simulink model "ALL_JP360_DBW_V6_5_1103"  (R2022a)
settings: Solver=FixedStepAuto  StartTime=0.0  StopTime=inf  FixedStep=0.01  RelTol=1e-3  EnableMultiTasking=on
model workspace (MAT data in the model file):
  g = 9.8
undefined symbols (not defined in the file or in its folder): canChannel, delta_v_p, IPM_Line_C0, IPM_Line_C1, IPM_Line_C2, IPM_Line_C3, M, M_p, MRR_ObjDistX, MRR_ObjDistY, MRR_ObjFusionCamID, MRR_ObjFusionSig, MRR_ObjID, MRR_ObjRelVelX, MRR_ObjRelVelY, MRR_ObjType, MRR_ObjUpdFlg, none, obj_vaild, untracktime, V, videoinput
libraries: canfdmsglib x230, canfdlib x76, slpidlib x24, simulink x18, dspstat3 x14, ctrlSharedLib x1, simulink_extras x1, imaqlib x1, realtime_pacer_lib x1, dspvision x1, visionsinks x1
(part 18 of 55)

== system ALL_JP360_DBW_V6_5_1103/MsgFromCAN/SRR_ADCU_MsgFromCAN/SRR_ADCU_FLR_OBJPos13_0x19D ==
  SRR_ADCU_FLR_OBJPos13_0x19DFromInData : Inport  OutDataTypeStr=Bus:CAN_FD_MESSAGE_BUS
  Bus Creator : BusCreator  Inputs=42  OutDataTypeStr=Bus:SRR_ADCU_FLR_OBJPos13_0x19D  NonVirtualBus=on
  CAN FD Unpack : canfdmsglib/CAN FD Unpack  CANdbFile=V363 SRR Private CAN-V1.3.dbc  MsgList=(none)  MsgName=FLR_OBJPos13_0x19D  ProtocolMode=CAN FD  MsgIDType=Standard (11-bit identifier)  MsgIdentifier=413  MsgLength=48  SignalInfo={'FLR_CRCCheck_0x19D','376','16','BE','unsigned','Standard','0','1','0','0','65535';'FLR_OBJ25_Dx','79','13','BE','unsigned','Standard','0','0.0625','-256','-256','255.938';'FLR_OBJ25_Dy','60','11','BE','unsigned','Standard','0','0.125','-128','-128','127.875';'FLR_OBJ25_ExistProb','112','6','BE','unsigned','Standard','0','2','0','0','100';'FLR_OBJ25_HeadingAngle','55','10','BE','unsigned','Standard','0','0.01','-3.14','-3.14','3.14';'FLR_OBJ25_Height','26','9','BE','unsigned','Standard','0','0.01','0','0','5.11';'FLR_OBJ25_Length','33','9','BE','unsigned','Standard','0','0.05','0','0','25.5';'FLR_OBJ25_Measured','126','2','BE','unsigned','Standard','0','1','0','0','3';'FLR_OBJ25_Motion_Status','162','3','BE','unsigned','Standard','0','1','0','0','7';'FLR_OBJ25_ObstacleProb','120','6','BE','unsigned','Standard','0','2','0','0','100';'FLR_OBJ25_RefPointDx','144','13','BE','unsigned','Standard','0','0.0625','-256','-256','255.938';'FLR_OBJ25_RefPointDy','141','11','BE','unsigned','Standard','0','0.125','-128','-128','127.875';'FLR_OBJ25_RefPointLoc','157','3','BE','unsigned','Standard','0','1','0','0','7';'FLR_OBJ25_RelAx','118','9','BE','unsigned','Standard','0','0.0625','-16','-16','15.9375';'FLR_OBJ25_RelAy','111','10','BE','unsigned','Standard','0','0.03125','-16','-16','15.9688';'FLR_OBJ25_RelVx','89','12','BE','unsigned','Standard','0','0.0625','-128','-128','127.938';'FLR_OBJ25_RelVy','85','10','BE','unsigned','Standard','0','0.125','-64','-64','63.875';'FLR_OBJ25_Track_Age','165','8','BE','unsigned','Standard','0','1','0','0','255';'FLR_OBJ25_Track_ID','1','7','BE','unsigned','Standard','0','1','0','0','127';'FLR_OBJ25_Type','14','3','BE','unsigned','Standard','0','1','0','0','7';'FLR_OBJ25_Width','19','11','BE','unsigned','Standard','0','0.01','0','0','12';'FLR_OBJ26_Dx','247','13','BE','unsigned','Standard','0','0.0625','-256','-256','255.938';'FLR_OBJ26_Dy','228','11','BE','unsigned','Standard','0','0.125','-128','-128','127.875';'FLR_OBJ26_ExistProb','280','6','BE','unsigned','Standard','0','2','0','0','100';'FLR_OBJ26_HeadingAngle','223','10','BE','unsigned','Standard','0','0.01','-3.14','-3.14','3.14';'FLR_OBJ26_Height','194','9','BE','unsigned','Standard','0','0.01','0','0','5.11';'FLR_OBJ26_Length','201','9','BE','unsigned','Standard','0','0.05','0','0','25.5';'FLR_OBJ26_Measured','294','2','BE','unsigned','Standard','0','1','0','0','3';'FLR_OBJ26_Motion_Status','330','3','BE','unsigned','Standard','0','1','0','0','7';'FLR_OBJ26_ObstacleProb','288','6','BE','unsigned','Standard','0','2','0','0','100';'FLR_OBJ26_RefPointDx','312','13','BE','unsigned','Standard','0','0.0625','-256','-256','255.938';'FLR_OBJ26_RefPointDy','309','11','BE','unsigned','Standard','0','0.125','-128','-128','127.875';'FLR_OBJ26_RefPointLoc','325','3','BE','unsigned','Standard','0','1','0','0','7';'FLR_OBJ26_RelAx','286','9','BE','unsigned','Standard','0','0.0625','-16','-16','15.9375';'FLR_OBJ26_RelAy','279','10','BE','unsigned','Standard','0','0.03125','-16','-16','15.9688';'FLR_OBJ26_RelVx','257','12','BE','unsigned','Standard','0','0.0625','-128','-128','127.938';'FLR_OBJ26_RelVy','253','10','BE','unsigned','Standard','0','0.125','-64','-64','63.875';'FLR_OBJ26_Track_Age','333','8','BE','unsigned','Standard','0','1','0','0','255';'FLR_OBJ26_Track_ID','169','7','BE','unsigned','Standard','0','1','0','0','127';'FLR_OBJ26_Type','182','3','BE','unsigned','Standard','0','1','0','0','7';'FLR_OBJ26_Width','187','11','BE','unsigned','Standard','0','0.01','0','0','12';'FLR_RollingCounter_0x19D','360','4','BE','unsigned','Standard','0','1','0','0','15'}  IDPort=off  TimestampPort=off  ErrorPort=off  RemotePort=off  LengthPort=off  StatusPort=off  BRSPort=off  ESIPort=off  DLCPort=off  ApplyMinMax=off
      settings: SourceProductBaseCode=ME,XP,VN  DataFormat=CANdb specified signals
  Data Type Conversion1 : DataTypeConversion  OutDataTypeStr=uint16  SaturateOnIntegerOverflow=off  RndMeth=Floor
  Data Type Conversion{4,8..10,13,19..20,24,28..30,33,39..40,42} (15 alike) : DataTypeConversion  OutDataTypeStr=int8  SaturateOnIntegerOverflow=off  RndMeth=Floor
  Data Type Conversion{2..3,5..7,11..12,14..17,21..23,25..27,31..32,34..37,41} (24 alike) : DataTypeConversion  OutDataTypeStr=single  SaturateOnIntegerOverflow=off  RndMeth=Floor
  Data Type Conversion18 : DataTypeConversion  OutDataTypeStr=uint8  SaturateOnIntegerOverflow=off  RndMeth=Floor
  Data Type Conversion38 : DataTypeConversion  OutDataTypeStr=uint8  SaturateOnIntegerOverflow=off  RndMeth=Floor
  SRR_ADCU_FLR_OBJPos13_0x19DFromOutData : Outport  OutDataTypeStr=Bus:SRR_ADCU_FLR_OBJPos13_0x19D
  wires:
  CAN FD Unpack/1 -> Data Type Conversion1/1
  CAN FD Unpack/2 -> Data Type Conversion2/1
  CAN FD Unpack/3 -> Data Type Conversion3/1
  CAN FD Unpack/4 -> Data Type Conversion4/1
  CAN FD Unpack/5 -> Data Type Conversion5/1
  CAN FD Unpack/6 -> Data Type Conversion6/1
  CAN FD Unpack/7 -> Data Type Conversion7/1
  CAN FD Unpack/8 -> Data Type Conversion8/1
  CAN FD Unpack/9 -> Data Type Conversion9/1
  CAN FD Unpack/10 -> Data Type Conversion10/1
  CAN FD Unpack/11 -> Data Type Conversion11/1
  CAN FD Unpack/12 -> Data Type Conversion12/1
  CAN FD Unpack/13 -> Data Type Conversion13/1
  CAN FD Unpack/14 -> Data Type Conversion14/1
  CAN FD Unpack/15 -> Data Type Conversion15/1
  CAN FD Unpack/16 -> Data Type Conversion16/1
  CAN FD Unpack/17 -> Data Type Conversion17/1
  CAN FD Unpack/18 -> Data Type Conversion18/1
  CAN FD Unpack/19 -> Data Type Conversion19/1
  CAN FD Unpack/20 -> Data Type Conversion20/1
  CAN FD Unpack/21 -> Data Type Conversion21/1
  CAN FD Unpack/22 -> Data Type Conversion22/1
  CAN FD Unpack/23 -> Data Type Conversion23/1
  CAN FD Unpack/24 -> Data Type Conversion24/1
  CAN FD Unpack/25 -> Data Type Conversion25/1
  CAN FD Unpack/26 -> Data Type Conversion26/1
  CAN FD Unpack/27 -> Data Type Conversion27/1
  CAN FD Unpack/28 -> Data Type Conversion28/1
  CAN FD Unpack/29 -> Data Type Conversion29/1
  CAN FD Unpack/30 -> Data Type Conversion30/1
  CAN FD Unpack/31 -> Data Type Conversion31/1
  CAN FD Unpack/32 -> Data Type Conversion32/1
  CAN FD Unpack/33 -> Data Type Conversion33/1
  CAN FD Unpack/34 -> Data Type Conversion34/1
  CAN FD Unpack/35 -> Data Type Conversion35/1
  CAN FD Unpack/36 -> Data Type Conversion36/1
  CAN FD Unpack/37 -> Data Type Conversion37/1
  CAN FD Unpack/38 -> Data Type Conversion38/1
  CAN FD Unpack/39 -> Data Type Conversion39/1
  CAN FD Unpack/40 -> Data Type Conversion40/1
  CAN FD Unpack/41 -> Data Type Conversion41/1
  CAN FD Unpack/42 -> Data Type Conversion42/1
  Data Type Conversion1/1 -> Bus Creator/1  "FLR_CRCCheck_0x19D"
  Data Type Conversion2/1 -> Bus Creator/2  "FLR_OBJ25_Dx"
  Data Type Conversion3/1 -> Bus Creator/3  "FLR_OBJ25_Dy"
  Data Type Conversion4/1 -> Bus Creator/4  "FLR_OBJ25_ExistProb"
  Data Type Conversion5/1 -> Bus Creator/5  "FLR_OBJ25_HeadingAngle"
  Data Type Conversion6/1 -> Bus Creator/6  "FLR_OBJ25_Height"
  Data Type Conversion7/1 -> Bus Creator/7  "FLR_OBJ25_Length"
  Data Type Conversion8/1 -> Bus Creator/8  "FLR_OBJ25_Measured"
  Data Type Conversion9/1 -> Bus Creator/9  "FLR_OBJ25_Motion_Status"
  Data Type Conversion10/1 -> Bus Creator/10  "FLR_OBJ25_ObstacleProb"
  Data Type Conversion11/1 -> Bus Creator/11  "FLR_OBJ25_RefPointDx"
  Data Type Conversion12/1 -> Bus Creator/12  "FLR_OBJ25_RefPointDy"
  Data Type Conversion13/1 -> Bus Creator/13  "FLR_OBJ25_RefPointLoc"
  Data Type Conversion14/1 -> Bus Creator/14  "FLR_OBJ25_RelAx"
  Data Type Conversion15/1 -> Bus Creator/15  "FLR_OBJ25_RelAy"
  Data Type Conversion16/1 -> Bus Creator/16  "FLR_OBJ25_RelVx"
  Data Type Conversion17/1 -> Bus Creator/17  "FLR_OBJ25_RelVy"
  Data Type Conversion18/1 -> Bus Creator/18  "FLR_OBJ25_Track_Age"
  Data Type Conversion19/1 -> Bus Creator/19  "FLR_OBJ25_Track_ID"
  Data Type Conversion20/1 -> Bus Creator/20  "FLR_OBJ25_Type"
  Data Type Conversion21/1 -> Bus Creator/21  "FLR_OBJ25_Width"
  Data Type Conversion22/1 -> Bus Creator/22  "FLR_OBJ26_Dx"
  Data Type Conversion23/1 -> Bus Creator/23  "FLR_OBJ26_Dy"
  Data Type Conversion24/1 -> Bus Creator/24  "FLR_OBJ26_ExistProb"
  Data Type Conversion25/1 -> Bus Creator/25  "FLR_OBJ26_HeadingAngle"
  Data Type Conversion26/1 -> Bus Creator/26  "FLR_OBJ26_Height"
  Data Type Conversion27/1 -> Bus Creator/27  "FLR_OBJ26_Length"
  Data Type Conversion28/1 -> Bus Creator/28  "FLR_OBJ26_Measured"
  Data Type Conversion29/1 -> Bus Creator/29  "FLR_OBJ26_Motion_Status"
  Data Type Conversion30/1 -> Bus Creator/30  "FLR_OBJ26_ObstacleProb"
  Data Type Conversion31/1 -> Bus Creator/31  "FLR_OBJ26_RefPointDx"
  Data Type Conversion32/1 -> Bus Creator/32  "FLR_OBJ26_RefPointDy"
  Data Type Conversion33/1 -> Bus Creator/33  "FLR_OBJ26_RefPointLoc"
  Data Type Conversion34/1 -> Bus Creator/34  "FLR_OBJ26_RelAx"
  Data Type Conversion35/1 -> Bus Creator/35  "FLR_OBJ26_RelAy"
  Data Type Conversion36/1 -> Bus Creator/36  "FLR_OBJ26_RelVx"
  Data Type Conversion37/1 -> Bus Creator/37  "FLR_OBJ26_RelVy"
  Data Type Conversion38/1 -> Bus Creator/38  "FLR_OBJ26_Track_Age"
  Data Type Conversion39/1 -> Bus Creator/39  "FLR_OBJ26_Track_ID"
  Data Type Conversion40/1 -> Bus Creator/40  "FLR_OBJ26_Type"
  Data Type Conversion41/1 -> Bus Creator/41  "FLR_OBJ26_Width"
  Data Type Conversion42/1 -> Bus Creator/42  "FLR_RollingCounter_0x19D"
  Bus Creator/1 -> SRR_ADCU_FLR_OBJPos13_0x19DFromOutData/1  "SRR_ADCU_FLR_OBJPos13_0x19DFromOutData"
  SRR_ADCU_FLR_OBJPos13_0x19DFromInData/1 -> CAN FD Unpack/1  "SRR_ADCU_FLR_OBJPos13_0x19DFromInData"

== system ALL_JP360_DBW_V6_5_1103/MsgFromCAN/SRR_ADCU_MsgFromCAN/SRR_ADCU_FLR_OBJPos14_0x19E ==
  SRR_ADCU_FLR_OBJPos14_0x19EFromInData : Inport  OutDataTypeStr=Bus:CAN_FD_MESSAGE_BUS
  Bus Creator : BusCreator  Inputs=42  OutDataTypeStr=Bus:SRR_ADCU_FLR_OBJPos14_0x19E  NonVirtualBus=on
  CAN FD Unpack : canfdmsglib/CAN FD Unpack  CANdbFile=V363 SRR Private CAN-V1.3.dbc  MsgList=(none)  MsgName=FLR_OBJPos14_0x19E  ProtocolMode=CAN FD  MsgIDType=Standard (11-bit identifier)  MsgIdentifier=414  MsgLength=48  SignalInfo={'FLR_CRCCheck_0x19E','376','16','BE','unsigned','Standard','0','1','0','0','65535';'FLR_OBJ27_Dx','79','13','BE','unsigned','Standard','0','0.0625','-256','-256','255.938';'FLR_OBJ27_Dy','60','11','BE','unsigned','Standard','0','0.125','-128','-128','127.875';'FLR_OBJ27_ExistProb','112','6','BE','unsigned','Standard','0','2','0','0','100';'FLR_OBJ27_HeadingAngle','55','10','BE','unsigned','Standard','0','0.01','-3.14','-3.14','3.14';'FLR_OBJ27_Height','26','9','BE','unsigned','Standard','0','0.01','0','0','5.11';'FLR_OBJ27_Length','33','9','BE','unsigned','Standard','0','0.05','0','0','25.5';'FLR_OBJ27_Measured','126','2','BE','unsigned','Standard','0','1','0','0','3';'FLR_OBJ27_Motion_Status','162','3','BE','unsigned','Standard','0','1','0','0','7';'FLR_OBJ27_ObstacleProb','120','6','BE','unsigned','Standard','0','2','0','0','100';'FLR_OBJ27_RefPointDx','144','13','BE','unsigned','Standard','0','0.0625','-256','-256','255.938';'FLR_OBJ27_RefPointDy','141','11','BE','unsigned','Standard','0','0.125','-128','-128','127.875';'FLR_OBJ27_RefPointLoc','157','3','BE','unsigned','Standard','0','1','0','0','7';'FLR_OBJ27_RelAx','118','9','BE','unsigned','Standard','0','0.0625','-16','-16','15.9375';'FLR_OBJ27_RelAy','111','10','BE','unsigned','Standard','0','0.03125','-16','-16','15.9688';'FLR_OBJ27_RelVx','89','12','BE','unsigned','Standard','0','0.0625','-128','-128','127.938';'FLR_OBJ27_RelVy','85','10','BE','unsigned','Standard','0','0.125','-64','-64','63.875';'FLR_OBJ27_Track_Age','165','8','BE','unsigned','Standard','0','1','0','0','255';'FLR_OBJ27_Track_ID','1','7','BE','unsigned','Standard','0','1','0','0','127';'FLR_OBJ27_Type','14','3','BE','unsigned','Standard','0','1','0','0','7';'FLR_OBJ27_Width','19','11','BE','unsigned','Standard','0','0.01','0','0','12';'FLR_OBJ28_Dx','247','13','BE','unsigned','Standard','0','0.0625','-256','-256','255.938';'FLR_OBJ28_Dy','228','11','BE','unsigned','Standard','0','0.125','-128','-128','127.875';'FLR_OBJ28_ExistProb','280','6','BE','unsigned','Standard','0','2','0','0','100';'FLR_OBJ28_HeadingAngle','223','10','BE','unsigned','Standard','0','0.01','-3.14','-3.14','3.14';'FLR_OBJ28_Height','194','9','BE','unsigned','Standard','0','0.01','0','0','5.11';'FLR_OBJ28_Length','201','9','BE','unsigned','Standard','0','0.05','0','0','25.5';'FLR_OBJ28_Measured','294','2','BE','unsigned','Standard','0','1','0','0','3';'FLR_OBJ28_Motion_Status','330','3','BE','unsigned','Standard','0','1','0','0','7';'FLR_OBJ28_ObstacleProb','288','6','BE','unsigned','Standard','0','2','0','0','100';'FLR_OBJ28_RefPointDx','312','13','BE','unsigned','Standard','0','0.0625','-256','-256','255.938';'FLR_OBJ28_RefPointDy','309','11','BE','unsigned','Standard','0','0.125','-128','-128','127.875';'FLR_OBJ28_RefPointLoc','325','3','BE','unsigned','Standard','0','1','0','0','7';'FLR_OBJ28_RelAx','286','9','BE','unsigned','Standard','0','0.0625','-16','-16','15.9375';'FLR_OBJ28_RelAy','279','10','BE','unsigned','Standard','0','0.03125','-16','-16','15.9688';'FLR_OBJ28_RelVx','257','12','BE','unsigned','Standard','0','0.0625','-128','-128','127.938';'FLR_OBJ28_RelVy','253','10','BE','unsigned','Standard','0','0.125','-64','-64','63.875';'FLR_OBJ28_Track_Age','333','8','BE','unsigned','Standard','0','1','0','0','255';'FLR_OBJ28_Track_ID','169','7','BE','unsigned','Standard','0','1','0','0','127';'FLR_OBJ28_Type','182','3','BE','unsigned','Standard','0','1','0','0','7';'FLR_OBJ28_Width','187','11','BE','unsigned','Standard','0','0.01','0','0','12';'FLR_RollingCounter_0x19E','360','4','BE','unsigned','Standard','0','1','0','0','15'}  IDPort=off  TimestampPort=off  ErrorPort=off  RemotePort=off  LengthPort=off  StatusPort=off  BRSPort=off  ESIPort=off  DLCPort=off  ApplyMinMax=off
      settings: SourceProductBaseCode=ME,XP,VN  DataFormat=CANdb specified signals
  Data Type Conversion1 : DataTypeConversion  OutDataTypeStr=uint16  SaturateOnIntegerOverflow=off  RndMeth=Floor
  Data Type Conversion{4,8..10,13,19..20,24,28..30,33,39..40,42} (15 alike) : DataTypeConversion  OutDataTypeStr=int8  SaturateOnIntegerOverflow=off  RndMeth=Floor
  Data Type Conversion{2..3,5..7,11..12,14..17,21..23,25..27,31..32,34..37,41} (24 alike) : DataTypeConversion  OutDataTypeStr=single  SaturateOnIntegerOverflow=off  RndMeth=Floor
  Data Type Conversion18 : DataTypeConversion  OutDataTypeStr=uint8  SaturateOnIntegerOverflow=off  RndMeth=Floor
  Data Type Conversion38 : DataTypeConversion  OutDataTypeStr=uint8  SaturateOnIntegerOverflow=off  RndMeth=Floor
  SRR_ADCU_FLR_OBJPos14_0x19EFromOutData : Outport  OutDataTypeStr=Bus:SRR_ADCU_FLR_OBJPos14_0x19E
  wires:
  CAN FD Unpack/1 -> Data Type Conversion1/1
  CAN FD Unpack/2 -> Data Type Conversion2/1
  CAN FD Unpack/3 -> Data Type Conversion3/1
  CAN FD Unpack/4 -> Data Type Conversion4/1
  CAN FD Unpack/5 -> Data Type Conversion5/1
  CAN FD Unpack/6 -> Data Type Conversion6/1
  CAN FD Unpack/7 -> Data Type Conversion7/1
  CAN FD Unpack/8 -> Data Type Conversion8/1
  CAN FD Unpack/9 -> Data Type Conversion9/1
  CAN FD Unpack/10 -> Data Type Conversion10/1
  CAN FD Unpack/11 -> Data Type Conversion11/1
  CAN FD Unpack/12 -> Data Type Conversion12/1
  CAN FD Unpack/13 -> Data Type Conversion13/1
  CAN FD Unpack/14 -> Data Type Conversion14/1
  CAN FD Unpack/15 -> Data Type Conversion15/1
  CAN FD Unpack/16 -> Data Type Conversion16/1
  CAN FD Unpack/17 -> Data Type Conversion17/1
  CAN FD Unpack/18 -> Data Type Conversion18/1
  CAN FD Unpack/19 -> Data Type Conversion19/1
  CAN FD Unpack/20 -> Data Type Conversion20/1
  CAN FD Unpack/21 -> Data Type Conversion21/1
  CAN FD Unpack/22 -> Data Type Conversion22/1
  CAN FD Unpack/23 -> Data Type Conversion23/1
  CAN FD Unpack/24 -> Data Type Conversion24/1
  CAN FD Unpack/25 -> Data Type Conversion25/1
  CAN FD Unpack/26 -> Data Type Conversion26/1
  CAN FD Unpack/27 -> Data Type Conversion27/1
  CAN FD Unpack/28 -> Data Type Conversion28/1
  CAN FD Unpack/29 -> Data Type Conversion29/1
  CAN FD Unpack/30 -> Data Type Conversion30/1
  CAN FD Unpack/31 -> Data Type Conversion31/1
  CAN FD Unpack/32 -> Data Type Conversion32/1
  CAN FD Unpack/33 -> Data Type Conversion33/1
  CAN FD Unpack/34 -> Data Type Conversion34/1
  CAN FD Unpack/35 -> Data Type Conversion35/1
  CAN FD Unpack/36 -> Data Type Conversion36/1
  CAN FD Unpack/37 -> Data Type Conversion37/1
  CAN FD Unpack/38 -> Data Type Conversion38/1
  CAN FD Unpack/39 -> Data Type Conversion39/1
  CAN FD Unpack/40 -> Data Type Conversion40/1
  CAN FD Unpack/41 -> Data Type Conversion41/1
  CAN FD Unpack/42 -> Data Type Conversion42/1
  Data Type Conversion1/1 -> Bus Creator/1  "FLR_CRCCheck_0x19E"
  Data Type Conversion2/1 -> Bus Creator/2  "FLR_OBJ27_Dx"
  Data Type Conversion3/1 -> Bus Creator/3  "FLR_OBJ27_Dy"
  Data Type Conversion4/1 -> Bus Creator/4  "FLR_OBJ27_ExistProb"
  Data Type Conversion5/1 -> Bus Creator/5  "FLR_OBJ27_HeadingAngle"
  Data Type Conversion6/1 -> Bus Creator/6  "FLR_OBJ27_Height"
  Data Type Conversion7/1 -> Bus Creator/7  "FLR_OBJ27_Length"
  Data Type Conversion8/1 -> Bus Creator/8  "FLR_OBJ27_Measured"
  Data Type Conversion9/1 -> Bus Creator/9  "FLR_OBJ27_Motion_Status"
  Data Type Conversion10/1 -> Bus Creator/10  "FLR_OBJ27_ObstacleProb"
  Data Type Conversion11/1 -> Bus Creator/11  "FLR_OBJ27_RefPointDx"
  Data Type Conversion12/1 -> Bus Creator/12  "FLR_OBJ27_RefPointDy"
  Data Type Conversion13/1 -> Bus Creator/13  "FLR_OBJ27_RefPointLoc"
  Data Type Conversion14/1 -> Bus Creator/14  "FLR_OBJ27_RelAx"
  Data Type Conversion15/1 -> Bus Creator/15  "FLR_OBJ27_RelAy"
  Data Type Conversion16/1 -> Bus Creator/16  "FLR_OBJ27_RelVx"
  Data Type Conversion17/1 -> Bus Creator/17  "FLR_OBJ27_RelVy"
  Data Type Conversion18/1 -> Bus Creator/18  "FLR_OBJ27_Track_Age"
  Data Type Conversion19/1 -> Bus Creator/19  "FLR_OBJ27_Track_ID"
  Data Type Conversion20/1 -> Bus Creator/20  "FLR_OBJ27_Type"
  Data Type Conversion21/1 -> Bus Creator/21  "FLR_OBJ27_Width"
  Data Type Conversion22/1 -> Bus Creator/22  "FLR_OBJ28_Dx"
  Data Type Conversion23/1 -> Bus Creator/23  "FLR_OBJ28_Dy"
  Data Type Conversion24/1 -> Bus Creator/24  "FLR_OBJ28_ExistProb"
  Data Type Conversion25/1 -> Bus Creator/25  "FLR_OBJ28_HeadingAngle"
  Data Type Conversion26/1 -> Bus Creator/26  "FLR_OBJ28_Height"
  Data Type Conversion27/1 -> Bus Creator/27  "FLR_OBJ28_Length"
  Data Type Conversion28/1 -> Bus Creator/28  "FLR_OBJ28_Measured"
  Data Type Conversion29/1 -> Bus Creator/29  "FLR_OBJ28_Motion_Status"
  Data Type Conversion30/1 -> Bus Creator/30  "FLR_OBJ28_ObstacleProb"
  Data Type Conversion31/1 -> Bus Creator/31  "FLR_OBJ28_RefPointDx"
  Data Type Conversion32/1 -> Bus Creator/32  "FLR_OBJ28_RefPointDy"
  Data Type Conversion33/1 -> Bus Creator/33  "FLR_OBJ28_RefPointLoc"
  Data Type Conversion34/1 -> Bus Creator/34  "FLR_OBJ28_RelAx"
  Data Type Conversion35/1 -> Bus Creator/35  "FLR_OBJ28_RelAy"
  Data Type Conversion36/1 -> Bus Creator/36  "FLR_OBJ28_RelVx"
  Data Type Conversion37/1 -> Bus Creator/37  "FLR_OBJ28_RelVy"
  Data Type Conversion38/1 -> Bus Creator/38  "FLR_OBJ28_Track_Age"
  Data Type Conversion39/1 -> Bus Creator/39  "FLR_OBJ28_Track_ID"
  Data Type Conversion40/1 -> Bus Creator/40  "FLR_OBJ28_Type"
  Data Type Conversion41/1 -> Bus Creator/41  "FLR_OBJ28_Width"
  Data Type Conversion42/1 -> Bus Creator/42  "FLR_RollingCounter_0x19E"
  Bus Creator/1 -> SRR_ADCU_FLR_OBJPos14_0x19EFromOutData/1  "SRR_ADCU_FLR_OBJPos14_0x19EFromOutData"
  SRR_ADCU_FLR_OBJPos14_0x19EFromInData/1 -> CAN FD Unpack/1  "SRR_ADCU_FLR_OBJPos14_0x19EFromInData"

== system ALL_JP360_DBW_V6_5_1103/MsgFromCAN/SRR_ADCU_MsgFromCAN/SRR_ADCU_FLR_OBJPos15_0x1A1 ==
  SRR_ADCU_FLR_OBJPos15_0x1A1FromInData : Inport  OutDataTypeStr=Bus:CAN_FD_MESSAGE_BUS
  Bus Creator : BusCreator  Inputs=42  OutDataTypeStr=Bus:SRR_ADCU_FLR_OBJPos15_0x1A1  NonVirtualBus=on
  CAN FD Unpack : canfdmsglib/CAN FD Unpack  CANdbFile=V363 SRR Private CAN-V1.3.dbc  MsgList=(none)  MsgName=FLR_OBJPos15_0x1A1  ProtocolMode=CAN FD  MsgIDType=Standard (11-bit identifier)  MsgIdentifier=417  MsgLength=48  SignalInfo={'FLR_CRCCheck_0x1A1','376','16','BE','unsigned','Standard','0','1','0','0','65535';'FLR_OBJ29_Dx','79','13','BE','unsigned','Standard','0','0.0625','-256','-256','255.938';'FLR_OBJ29_Dy','60','11','BE','unsigned','Standard','0','0.125','-128','-128','127.875';'FLR_OBJ29_ExistProb','112','6','BE','unsigned','Standard','0','2','0','0','100';'FLR_OBJ29_HeadingAngle','55','10','BE','unsigned','Standard','0','0.01','-3.14','-3.14','3.14';'FLR_OBJ29_Height','26','9','BE','unsigned','Standard','0','0.01','0','0','5.11';'FLR_OBJ29_Length','33','9','BE','unsigned','Standard','0','0.05','0','0','25.5';'FLR_OBJ29_Measured','126','2','BE','unsigned','Standard','0','1','0','0','3';'FLR_OBJ29_Motion_Status','162','3','BE','unsigned','Standard','0','1','0','0','7';'FLR_OBJ29_ObstacleProb','120','6','BE','unsigned','Standard','0','2','0','0','100';'FLR_OBJ29_RefPointDx','144','13','BE','unsigned','Standard','0','0.0625','-256','-256','255.938';'FLR_OBJ29_RefPointDy','141','11','BE','unsigned','Standard','0','0.125','-128','-128','127.875';'FLR_OBJ29_RefPointLoc','157','3','BE','unsigned','Standard','0','1','0','0','7';'FLR_OBJ29_RelAx','118','9','BE','unsigned','Standard','0','0.0625','-16','-16','15.9375';'FLR_OBJ29_RelAy','111','10','BE','unsigned','Standard','0','0.03125','-16','-16','15.9688';'FLR_OBJ29_RelVx','89','12','BE','unsigned','Standard','0','0.0625','-128','-128','127.938';'FLR_OBJ29_RelVy','85','10','BE','unsigned','Standard','0','0.125','-64','-64','63.875';'FLR_OBJ29_Track_Age','165','8','BE','unsigned','Standard','0','1','0','0','255';'FLR_OBJ29_Track_ID','1','7','BE','unsigned','Standard','0','1','0','0','127';'FLR_OBJ29_Type','14','3','BE','unsigned','Standard','0','1','0','0','7';'FLR_OBJ29_Width','19','11','BE','unsigned','Standard','0','0.01','0','0','12';'FLR_OBJ30_Dx','247','13','BE','unsigned','Standard','0','0.0625','-256','-256','255.938';'FLR_OBJ30_Dy','228','11','BE','unsigned','Standard','0','0.125','-128','-128','127.875';'FLR_OBJ30_ExistProb','280','6','BE','unsigned','Standard','0','2','0','0','100';'FLR_OBJ30_HeadingAngle','223','10','BE','unsigned','Standard','0','0.01','-3.14','-3.14','3.14';'FLR_OBJ30_Height','194','9','BE','unsigned','Standard','0','0.01','0','0','5.11';'FLR_OBJ30_Length','201','9','BE','unsigned','Standard','0','0.05','0','0','25.5';'FLR_OBJ30_Measured','294','2','BE','unsigned','Standard','0','1','0','0','3';'FLR_OBJ30_Motion_Status','330','3','BE','unsigned','Standard','0','1','0','0','7';'FLR_OBJ30_ObstacleProb','288','6','BE','unsigned','Standard','0','2','0','0','100';'FLR_OBJ30_RefPointDx','312','13','BE','unsigned','Standard','0','0.0625','-256','-256','255.938';'FLR_OBJ30_RefPointDy','309','11','BE','unsigned','Standard','0','0.125','-128','-128','127.875';'FLR_OBJ30_RefPointLoc','325','3','BE','unsigned','Standard','0','1','0','0','7';'FLR_OBJ30_RelAx','286','9','BE','unsigned','Standard','0','0.0625','-16','-16','15.9375';'FLR_OBJ30_RelAy','279','10','BE','unsigned','Standard','0','0.03125','-16','-16','15.9688';'FLR_OBJ30_RelVx','257','12','BE','unsigned','Standard','0','0.0625','-128','-128','127.938';'FLR_OBJ30_RelVy','253','10','BE','unsigned','Standard','0','0.125','-64','-64','63.875';'FLR_OBJ30_Track_Age','333','8','BE','unsigned','Standard','0','1','0','0','255';'FLR_OBJ30_Track_ID','169','7','BE','unsigned','Standard','0','1','0','0','127';'FLR_OBJ30_Type','182','3','BE','unsigned','Standard','0','1','0','0','7';'FLR_OBJ30_Width','187','11','BE','unsigned','Standard','0','0.01','0','0','12';'FLR_RollingCounter_0x1A1','360','4','BE','unsigned','Standard','0','1','0','0','15'}  IDPort=off  TimestampPort=off  ErrorPort=off  RemotePort=off  LengthPort=off  StatusPort=off  BRSPort=off  ESIPort=off  DLCPort=off  ApplyMinMax=off
      settings: SourceProductBaseCode=ME,XP,VN  DataFormat=CANdb specified signals
  Data Type Conversion1 : DataTypeConversion  OutDataTypeStr=uint16  SaturateOnIntegerOverflow=off  RndMeth=Floor
  Data Type Conversion{4,8..10,13,19..20,24,28..30,33,39..40,42} (15 alike) : DataTypeConversion  OutDataTypeStr=int8  SaturateOnIntegerOverflow=off  RndMeth=Floor
  Data Type Conversion{2..3,5..7,11..12,14..17,21..23,25..27,31..32,34..37,41} (24 alike) : DataTypeConversion  OutDataTypeStr=single  SaturateOnIntegerOverflow=off  RndMeth=Floor
  Data Type Conversion18 : DataTypeConversion  OutDataTypeStr=uint8  SaturateOnIntegerOverflow=off  RndMeth=Floor
  Data Type Conversion38 : DataTypeConversion  OutDataTypeStr=uint8  SaturateOnIntegerOverflow=off  RndMeth=Floor
  SRR_ADCU_FLR_OBJPos15_0x1A1FromOutData : Outport  OutDataTypeStr=Bus:SRR_ADCU_FLR_OBJPos15_0x1A1
  wires:
  CAN FD Unpack/1 -> Data Type Conversion1/1
  CAN FD Unpack/2 -> Data Type Conversion2/1
  CAN FD Unpack/3 -> Data Type Conversion3/1
  CAN FD Unpack/4 -> Data Type Conversion4/1
  CAN FD Unpack/5 -> Data Type Conversion5/1
  CAN FD Unpack/6 -> Data Type Conversion6/1
  CAN FD Unpack/7 -> Data Type Conversion7/1
  CAN FD Unpack/8 -> Data Type Conversion8/1
  CAN FD Unpack/9 -> Data Type Conversion9/1
  CAN FD Unpack/10 -> Data Type Conversion10/1
  CAN FD Unpack/11 -> Data Type Conversion11/1
  CAN FD Unpack/12 -> Data Type Conversion12/1
  CAN FD Unpack/13 -> Data Type Conversion13/1
  CAN FD Unpack/14 -> Data Type Conversion14/1
  CAN FD Unpack/15 -> Data Type Conversion15/1
  CAN FD Unpack/16 -> Data Type Conversion16/1
  CAN FD Unpack/17 -> Data Type Conversion17/1
  CAN FD Unpack/18 -> Data Type Conversion18/1
  CAN FD Unpack/19 -> Data Type Conversion19/1
  CAN FD Unpack/20 -> Data Type Conversion20/1
  CAN FD Unpack/21 -> Data Type Conversion21/1
  CAN FD Unpack/22 -> Data Type Conversion22/1
  CAN FD Unpack/23 -> Data Type Conversion23/1
  CAN FD Unpack/24 -> Data Type Conversion24/1
  CAN FD Unpack/25 -> Data Type Conversion25/1
  CAN FD Unpack/26 -> Data Type Conversion26/1
  CAN FD Unpack/27 -> Data Type Conversion27/1
  CAN FD Unpack/28 -> Data Type Conversion28/1
  CAN FD Unpack/29 -> Data Type Conversion29/1
  CAN FD Unpack/30 -> Data Type Conversion30/1
  CAN FD Unpack/31 -> Data Type Conversion31/1
  CAN FD Unpack/32 -> Data Type Conversion32/1
  CAN FD Unpack/33 -> Data Type Conversion33/1
  CAN FD Unpack/34 -> Data Type Conversion34/1
  CAN FD Unpack/35 -> Data Type Conversion35/1
  CAN FD Unpack/36 -> Data Type Conversion36/1
  CAN FD Unpack/37 -> Data Type Conversion37/1
  CAN FD Unpack/38 -> Data Type Conversion38/1
  CAN FD Unpack/39 -> Data Type Conversion39/1
  CAN FD Unpack/40 -> Data Type Conversion40/1
  CAN FD Unpack/41 -> Data Type Conversion41/1
  CAN FD Unpack/42 -> Data Type Conversion42/1
  Data Type Conversion1/1 -> Bus Creator/1  "FLR_CRCCheck_0x1A1"
  Data Type Conversion2/1 -> Bus Creator/2  "FLR_OBJ29_Dx"
  Data Type Conversion3/1 -> Bus Creator/3  "FLR_OBJ29_Dy"
  Data Type Conversion4/1 -> Bus Creator/4  "FLR_OBJ29_ExistProb"
  Data Type Conversion5/1 -> Bus Creator/5  "FLR_OBJ29_HeadingAngle"
  Data Type Conversion6/1 -> Bus Creator/6  "FLR_OBJ29_Height"
  Data Type Conversion7/1 -> Bus Creator/7  "FLR_OBJ29_Length"
  Data Type Conversion8/1 -> Bus Creator/8  "FLR_OBJ29_Measured"
  Data Type Conversion9/1 -> Bus Creator/9  "FLR_OBJ29_Motion_Status"
  Data Type Conversion10/1 -> Bus Creator/10  "FLR_OBJ29_ObstacleProb"
  Data Type Conversion11/1 -> Bus Creator/11  "FLR_OBJ29_RefPointDx"
  Data Type Conversion12/1 -> Bus Creator/12  "FLR_OBJ29_RefPointDy"
  Data Type Conversion13/1 -> Bus Creator/13  "FLR_OBJ29_RefPointLoc"
  Data Type Conversion14/1 -> Bus Creator/14  "FLR_OBJ29_RelAx"
  Data Type Conversion15/1 -> Bus Creator/15  "FLR_OBJ29_RelAy"
  Data Type Conversion16/1 -> Bus Creator/16  "FLR_OBJ29_RelVx"
  Data Type Conversion17/1 -> Bus Creator/17  "FLR_OBJ29_RelVy"
  Data Type Conversion18/1 -> Bus Creator/18  "FLR_OBJ29_Track_Age"
  Data Type Conversion19/1 -> Bus Creator/19  "FLR_OBJ29_Track_ID"
  Data Type Conversion20/1 -> Bus Creator/20  "FLR_OBJ29_Type"
  Data Type Conversion21/1 -> Bus Creator/21  "FLR_OBJ29_Width"
  Data Type Conversion22/1 -> Bus Creator/22  "FLR_OBJ30_Dx"
  Data Type Conversion23/1 -> Bus Creator/23  "FLR_OBJ30_Dy"
  Data Type Conversion24/1 -> Bus Creator/24  "FLR_OBJ30_ExistProb"
  Data Type Conversion25/1 -> Bus Creator/25  "FLR_OBJ30_HeadingAngle"
  Data Type Conversion26/1 -> Bus Creator/26  "FLR_OBJ30_Height"
  Data Type Conversion27/1 -> Bus Creator/27  "FLR_OBJ30_Length"
  Data Type Conversion28/1 -> Bus Creator/28  "FLR_OBJ30_Measured"
  Data Type Conversion29/1 -> Bus Creator/29  "FLR_OBJ30_Motion_Status"
  Data Type Conversion30/1 -> Bus Creator/30  "FLR_OBJ30_ObstacleProb"
  Data Type Conversion31/1 -> Bus Creator/31  "FLR_OBJ30_RefPointDx"
  Data Type Conversion32/1 -> Bus Creator/32  "FLR_OBJ30_RefPointDy"
  Data Type Conversion33/1 -> Bus Creator/33  "FLR_OBJ30_RefPointLoc"
  Data Type Conversion34/1 -> Bus Creator/34  "FLR_OBJ30_RelAx"
  Data Type Conversion35/1 -> Bus Creator/35  "FLR_OBJ30_RelAy"
  Data Type Conversion36/1 -> Bus Creator/36  "FLR_OBJ30_RelVx"
  Data Type Conversion37/1 -> Bus Creator/37  "FLR_OBJ30_RelVy"
  Data Type Conversion38/1 -> Bus Creator/38  "FLR_OBJ30_Track_Age"
  Data Type Conversion39/1 -> Bus Creator/39  "FLR_OBJ30_Track_ID"
  Data Type Conversion40/1 -> Bus Creator/40  "FLR_OBJ30_Type"
  Data Type Conversion41/1 -> Bus Creator/41  "FLR_OBJ30_Width"
  Data Type Conversion42/1 -> Bus Creator/42  "FLR_RollingCounter_0x1A1"
  Bus Creator/1 -> SRR_ADCU_FLR_OBJPos15_0x1A1FromOutData/1  "SRR_ADCU_FLR_OBJPos15_0x1A1FromOutData"
  SRR_ADCU_FLR_OBJPos15_0x1A1FromInData/1 -> CAN FD Unpack/1  "SRR_ADCU_FLR_OBJPos15_0x1A1FromInData"

== system ALL_JP360_DBW_V6_5_1103/MsgFromCAN/SRR_ADCU_MsgFromCAN/SRR_ADCU_FLR_OBJPos16_0x1A2 ==
  SRR_ADCU_FLR_OBJPos16_0x1A2FromInData : Inport  OutDataTypeStr=Bus:CAN_FD_MESSAGE_BUS
  Bus Creator : BusCreator  Inputs=42  OutDataTypeStr=Bus:SRR_ADCU_FLR_OBJPos16_0x1A2  NonVirtualBus=on
  CAN FD Unpack : canfdmsglib/CAN FD Unpack  CANdbFile=V363 SRR Private CAN-V1.3.dbc  MsgList=(none)  MsgName=FLR_OBJPos16_0x1A2  ProtocolMode=CAN FD  MsgIDType=Standard (11-bit identifier)  MsgIdentifier=418  MsgLength=48  SignalInfo={'FLR_CRCCheck_0x1A2','376','16','BE','unsigned','Standard','0','1','0','0','65535';'FLR_OBJ31_Dx','79','13','BE','unsigned','Standard','0','0.0625','-256','-256','255.938';'FLR_OBJ31_Dy','60','11','BE','unsigned','Standard','0','0.125','-128','-128','127.875';'FLR_OBJ31_ExistProb','112','6','BE','unsigned','Standard','0','2','0','0','100';'FLR_OBJ31_HeadingAngle','55','10','BE','unsigned','Standard','0','0.01','-3.14','-3.14','3.14';'FLR_OBJ31_Height','26','9','BE','unsigned','Standard','0','0.01','0','0','5.11';'FLR_OBJ31_Length','33','9','BE','unsigned','Standard','0','0.05','0','0','25.5';'FLR_OBJ31_Measured','126','2','BE','unsigned','Standard','0','1','0','0','3';'FLR_OBJ31_Motion_Status','162','3','BE','unsigned','Standard','0','1','0','0','7';'FLR_OBJ31_ObstacleProb','120','6','BE','unsigned','Standard','0','2','0','0','100';'FLR_OBJ31_RefPointDx','144','13','BE','unsigned','Standard','0','0.0625','-256','-256','255.938';'FLR_OBJ31_RefPointDy','141','11','BE','unsigned','Standard','0','0.125','-128','-128','127.875';'FLR_OBJ31_RefPointLoc','157','3','BE','unsigned','Standard','0','1','0','0','7';'FLR_OBJ31_RelAx','118','9','BE','unsigned','Standard','0','0.0625','-16','-16','15.9375';'FLR_OBJ31_RelAy','111','10','BE','unsigned','Standard','0','0.03125','-16','-16','15.9688';'FLR_OBJ31_RelVx','89','12','BE','unsigned','Standard','0','0.0625','-128','-128','127.938';'FLR_OBJ31_RelVy','85','10','BE','unsigned','Standard','0','0.125','-64','-64','63.875';'FLR_OBJ31_Track_Age','165','8','BE','unsigned','Standard','0','1','0','0','255';'FLR_OBJ31_Track_ID','1','7','BE','unsigned','Standard','0','1','0','0','127';'FLR_OBJ31_Type','14','3','BE','unsigned','Standard','0','1','0','0','7';'FLR_OBJ31_Width','19','11','BE','unsigned','Standard','0','0.01','0','0','12';'FLR_OBJ32_Dx','247','13','BE','unsigned','Standard','0','0.0625','-256','-256','255.938';'FLR_OBJ32_Dy','228','11','BE','unsigned','Standard','0','0.125','-128','-128','127.875';'FLR_OBJ32_ExistProb','280','6','BE','unsigned','Standard','0','2','0','0','100';'FLR_OBJ32_HeadingAngle','223','10','BE','unsigned','Standard','0','0.01','-3.14','-3.14','3.14';'FLR_OBJ32_Height','194','9','BE','unsigned','Standard','0','0.01','0','0','5.11';'FLR_OBJ32_Length','201','9','BE','unsigned','Standard','0','0.05','0','0','25.5';'FLR_OBJ32_Measured','294','2','BE','unsigned','Standard','0','1','0','0','3';'FLR_OBJ32_Motion_Status','330','3','BE','unsigned','Standard','0','1','0','0','7';'FLR_OBJ32_ObstacleProb','288','6','BE','unsigned','Standard','0','2','0','0','100';'FLR_OBJ32_RefPointDx','312','13','BE','unsigned','Standard','0','0.0625','-256','-256','255.938';'FLR_OBJ32_RefPointDy','309','11','BE','unsigned','Standard','0','0.125','-128','-128','127.875';'FLR_OBJ32_RefPointLoc','325','3','BE','unsigned','Standard','0','1','0','0','7';'FLR_OBJ32_RelAx','286','9','BE','unsigned','Standard','0','0.0625','-16','-16','15.9375';'FLR_OBJ32_RelAy','279','10','BE','unsigned','Standard','0','0.03125','-16','-16','15.9688';'FLR_OBJ32_RelVx','257','12','BE','unsigned','Standard','0','0.0625','-128','-128','127.938';'FLR_OBJ32_RelVy','253','10','BE','unsigned','Standard','0','0.125','-64','-64','63.875';'FLR_OBJ32_Track_Age','333','8','BE','unsigned','Standard','0','1','0','0','255';'FLR_OBJ32_Track_ID','169','7','BE','unsigned','Standard','0','1','0','0','127';'FLR_OBJ32_Type','182','3','BE','unsigned','Standard','0','1','0','0','7';'FLR_OBJ32_Width','187','11','BE','unsigned','Standard','0','0.01','0','0','12';'FLR_RollingCounter_0x1A2','360','4','BE','unsigned','Standard','0','1','0','0','15'}  IDPort=off  TimestampPort=off  ErrorPort=off  RemotePort=off  LengthPort=off  StatusPort=off  BRSPort=off  ESIPort=off  DLCPort=off  ApplyMinMax=off
      settings: SourceProductBaseCode=ME,XP,VN  DataFormat=CANdb specified signals
  Data Type Conversion1 : DataTypeConversion  OutDataTypeStr=uint16  SaturateOnIntegerOverflow=off  RndMeth=Floor
  Data Type Conversion{4,8..10,13,19..20,24,28..30,33,39..40,42} (15 alike) : DataTypeConversion  OutDataTypeStr=int8  SaturateOnIntegerOverflow=off  RndMeth=Floor
  Data Type Conversion{2..3,5..7,11..12,14..17,21..23,25..27,31..32,34..37,41} (24 alike) : DataTypeConversion  OutDataTypeStr=single  SaturateOnIntegerOverflow=off  RndMeth=Floor
  Data Type Conversion18 : DataTypeConversion  OutDataTypeStr=uint8  SaturateOnIntegerOverflow=off  RndMeth=Floor
  Data Type Conversion38 : DataTypeConversion  OutDataTypeStr=uint8  SaturateOnIntegerOverflow=off  RndMeth=Floor
  SRR_ADCU_FLR_OBJPos16_0x1A2FromOutData : Outport  OutDataTypeStr=Bus:SRR_ADCU_FLR_OBJPos16_0x1A2
  wires:
  CAN FD Unpack/1 -> Data Type Conversion1/1
  CAN FD Unpack/2 -> Data Type Conversion2/1
  CAN FD Unpack/3 -> Data Type Conversion3/1
  CAN FD Unpack/4 -> Data Type Conversion4/1
  CAN FD Unpack/5 -> Data Type Conversion5/1
  CAN FD Unpack/6 -> Data Type Conversion6/1
  CAN FD Unpack/7 -> Data Type Conversion7/1
  CAN FD Unpack/8 -> Data Type Conversion8/1
  CAN FD Unpack/9 -> Data Type Conversion9/1
  CAN FD Unpack/10 -> Data Type Conversion10/1
  CAN FD Unpack/11 -> Data Type Conversion11/1
  CAN FD Unpack/12 -> Data Type Conversion12/1
  CAN FD Unpack/13 -> Data Type Conversion13/1
  CAN FD Unpack/14 -> Data Type Conversion14/1
  CAN FD Unpack/15 -> Data Type Conversion15/1
  CAN FD Unpack/16 -> Data Type Conversion16/1
  CAN FD Unpack/17 -> Data Type Conversion17/1
  CAN FD Unpack/18 -> Data Type Conversion18/1
  CAN FD Unpack/19 -> Data Type Conversion19/1
  CAN FD Unpack/20 -> Data Type Conversion20/1
  CAN FD Unpack/21 -> Data Type Conversion21/1
  CAN FD Unpack/22 -> Data Type Conversion22/1
  CAN FD Unpack/23 -> Data Type Conversion23/1
  CAN FD Unpack/24 -> Data Type Conversion24/1
  CAN FD Unpack/25 -> Data Type Conversion25/1
  CAN FD Unpack/26 -> Data Type Conversion26/1
  CAN FD Unpack/27 -> Data Type Conversion27/1
  CAN FD Unpack/28 -> Data Type Conversion28/1
  CAN FD Unpack/29 -> Data Type Conversion29/1
  CAN FD Unpack/30 -> Data Type Conversion30/1
  CAN FD Unpack/31 -> Data Type Conversion31/1
  CAN FD Unpack/32 -> Data Type Conversion32/1
  CAN FD Unpack/33 -> Data Type Conversion33/1
  CAN FD Unpack/34 -> Data Type Conversion34/1
  CAN FD Unpack/35 -> Data Type Conversion35/1
  CAN FD Unpack/36 -> Data Type Conversion36/1
  CAN FD Unpack/37 -> Data Type Conversion37/1
  CAN FD Unpack/38 -> Data Type Conversion38/1
  CAN FD Unpack/39 -> Data Type Conversion39/1
  CAN FD Unpack/40 -> Data Type Conversion40/1
  CAN FD Unpack/41 -> Data Type Conversion41/1
  CAN FD Unpack/42 -> Data Type Conversion42/1
  Data Type Conversion1/1 -> Bus Creator/1  "FLR_CRCCheck_0x1A2"
  Data Type Conversion2/1 -> Bus Creator/2  "FLR_OBJ31_Dx"
  Data Type Conversion3/1 -> Bus Creator/3  "FLR_OBJ31_Dy"
  Data Type Conversion4/1 -> Bus Creator/4  "FLR_OBJ31_ExistProb"
  Data Type Conversion5/1 -> Bus Creator/5  "FLR_OBJ31_HeadingAngle"
  Data Type Conversion6/1 -> Bus Creator/6  "FLR_OBJ31_Height"
  Data Type Conversion7/1 -> Bus Creator/7  "FLR_OBJ31_Length"
  Data Type Conversion8/1 -> Bus Creator/8  "FLR_OBJ31_Measured"
  Data Type Conversion9/1 -> Bus Creator/9  "FLR_OBJ31_Motion_Status"
  Data Type Conversion10/1 -> Bus Creator/10  "FLR_OBJ31_ObstacleProb"
  Data Type Conversion11/1 -> Bus Creator/11  "FLR_OBJ31_RefPointDx"
  Data Type Conversion12/1 -> Bus Creator/12  "FLR_OBJ31_RefPointDy"
  Data Type Conversion13/1 -> Bus Creator/13  "FLR_OBJ31_RefPointLoc"
  Data Type Conversion14/1 -> Bus Creator/14  "FLR_OBJ31_RelAx"
  Data Type Conversion15/1 -> Bus Creator/15  "FLR_OBJ31_RelAy"
  Data Type Conversion16/1 -> Bus Creator/16  "FLR_OBJ31_RelVx"
  Data Type Conversion17/1 -> Bus Creator/17  "FLR_OBJ31_RelVy"
  Data Type Conversion18/1 -> Bus Creator/18  "FLR_OBJ31_Track_Age"
  Data Type Conversion19/1 -> Bus Creator/19  "FLR_OBJ31_Track_ID"
  Data Type Conversion20/1 -> Bus Creator/20  "FLR_OBJ31_Type"
  Data Type Conversion21/1 -> Bus Creator/21  "FLR_OBJ31_Width"
  Data Type Conversion22/1 -> Bus Creator/22  "FLR_OBJ32_Dx"
  Data Type Conversion23/1 -> Bus Creator/23  "FLR_OBJ32_Dy"
  Data Type Conversion24/1 -> Bus Creator/24  "FLR_OBJ32_ExistProb"
  Data Type Conversion25/1 -> Bus Creator/25  "FLR_OBJ32_HeadingAngle"
  Data Type Conversion26/1 -> Bus Creator/26  "FLR_OBJ32_Height"
  Data Type Conversion27/1 -> Bus Creator/27  "FLR_OBJ32_Length"
  Data Type Conversion28/1 -> Bus Creator/28  "FLR_OBJ32_Measured"
  Data Type Conversion29/1 -> Bus Creator/29  "FLR_OBJ32_Motion_Status"
  Data Type Conversion30/1 -> Bus Creator/30  "FLR_OBJ32_ObstacleProb"
  Data Type Conversion31/1 -> Bus Creator/31  "FLR_OBJ32_RefPointDx"
  Data Type Conversion32/1 -> Bus Creator/32  "FLR_OBJ32_RefPointDy"
  Data Type Conversion33/1 -> Bus Creator/33  "FLR_OBJ32_RefPointLoc"
  Data Type Conversion34/1 -> Bus Creator/34  "FLR_OBJ32_RelAx"
  Data Type Conversion35/1 -> Bus Creator/35  "FLR_OBJ32_RelAy"
  Data Type Conversion36/1 -> Bus Creator/36  "FLR_OBJ32_RelVx"
  Data Type Conversion37/1 -> Bus Creator/37  "FLR_OBJ32_RelVy"
  Data Type Conversion38/1 -> Bus Creator/38  "FLR_OBJ32_Track_Age"
  Data Type Conversion39/1 -> Bus Creator/39  "FLR_OBJ32_Track_ID"
  Data Type Conversion40/1 -> Bus Creator/40  "FLR_OBJ32_Type"
  Data Type Conversion41/1 -> Bus Creator/41  "FLR_OBJ32_Width"
  Data Type Conversion42/1 -> Bus Creator/42  "FLR_RollingCounter_0x1A2"
  Bus Creator/1 -> SRR_ADCU_FLR_OBJPos16_0x1A2FromOutData/1  "SRR_ADCU_FLR_OBJPos16_0x1A2FromOutData"
  SRR_ADCU_FLR_OBJPos16_0x1A2FromInData/1 -> CAN FD Unpack/1  "SRR_ADCU_FLR_OBJPos16_0x1A2FromInData"
